simulink model "NewControlSim"  (R2024b)
settings: Solver=ode23s  StartTime=0.0  StopTime=173  RelTol=1e-3
values from neighbouring files (symbols this model uses):
  Af = 0.94    [new-sim-workspace.mat]    (also in workspace-var-complete-jan.mat; workspace_var_dec_2024.mat; workspace_var_jan_2024.mat)
  B = 10    [new-sim-workspace.mat]    (also in workspace-var-complete-jan.mat; workspace-vars.mat; workspace_var_dec_2024.mat; workspace_var_jan_2024.mat)
  C = 1.9    [new-sim-workspace.mat]    (also in workspace-var-complete-jan.mat; workspace-vars.mat; workspace_var_dec_2024.mat; workspace_var_jan_2024.mat)
  car_power_limit = 40    [new-sim-workspace.mat]    (also in workspace-var-complete-jan.mat)
  Cd = 0.94    [new-sim-workspace.mat]    (also in workspace-var-complete-jan.mat; workspace_var_dec_2024.mat; workspace_var_jan_2024.mat)
  cutoff_motor_temp = 90    [new-sim-workspace.mat]    (also in workspace-var-complete-jan.mat)
  D = 1    [new-sim-workspace.mat]    (also in workspace-var-complete-jan.mat; workspace-vars.mat; workspace_var_dec_2024.mat; workspace_var_jan_2024.mat)
  decrement_ratio_PL = 2.66666666667    [new-sim-workspace.mat]    (also in workspace-var-complete-jan.mat)
  g = 9.81    [new-sim-workspace.mat]    (also in workspace-var-complete-jan.mat; workspace-vars.mat; workspace_var_dec_2024.mat; workspace_var_jan_2024.mat)
  ideal_slip = 0.05    [new-sim-workspace.mat]    (also in workspace-var-complete-jan.mat)
  J_w = 0.5    [new-sim-workspace.mat]    (also in workspace-var-complete-jan.mat; workspace-vars.mat; workspace_var_dec_2024.mat; workspace_var_jan_2024.mat)
  M = 100    [new-sim-workspace.mat]    (also in workspace-var-complete-jan.mat; workspace-vars.mat; workspace_var_dec_2024.mat; workspace_var_jan_2024.mat)
  mass_den = 1.225    [new-sim-workspace.mat]    (also in workspace-var-complete-jan.mat; workspace_var_dec_2024.mat; workspace_var_jan_2024.mat)
  max_torque_req = 90    [new-sim-workspace.mat]    (also in workspace-var-complete-jan.mat)
  R = 0.5    [new-sim-workspace.mat]    (also in workspace-var-complete-jan.mat; workspace-vars.mat; workspace_var_dec_2024.mat; workspace_var_jan_2024.mat)
libraries: slpidlib x1
settings Model: Creator=shykizzy  LastModifiedBy=shykizzy

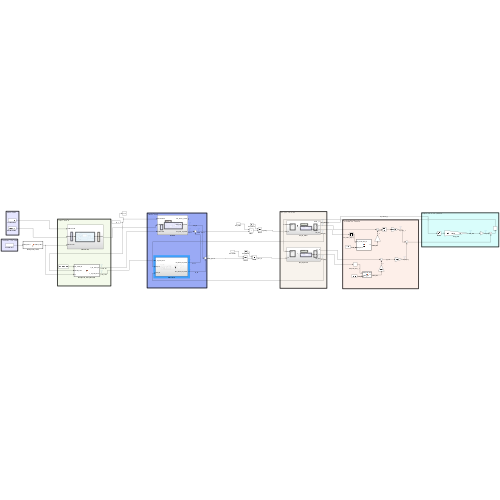
[thumbnail: Simulink's stored preview of the top-level diagram]
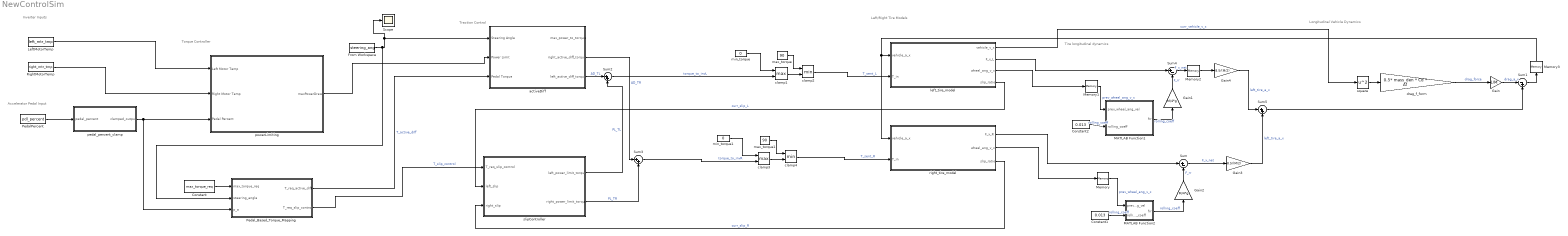
== system NewControlSim ==
  note: Longitudinal Vehicle Dynamics
  note: Traction Control
  note: Torque Controller
  note: Left/Right Tire Models
  note: Accelerator Pedal Input
  note: Inverter Inputs
  note: Tire longitudinal dynamics
  Constant : Constant  Value=max_torque_req
  Constant1 : Constant  Value=0.013
  Constant2 : Constant  Value=0.013
  From Workspace : FromWorkspace  VariableName=steering_ang
  Gain : Gain  Gain=1/M
  Gain1 : Gain  Gain=M/4*g
  Gain2 : Gain  Gain=M/4*g
  Gain3 : Gain  Gain=8.5/(M/2)
  Gain4 : Gain  Gain=8.5/(M/2)
  LeftMotorTemp : FromWorkspace  VariableName=left_mtr_tmp
  MATLAB Function1 : MATLAB Function  TreatAsAtomicUnit=on
  MATLAB Function2 : MATLAB Function  TreatAsAtomicUnit=on
  Memory{,1..3} (4 alike) : Memory
  PedalPercent : FromWorkspace  VariableName=pdl_percent
  Pedal_Based_Torque_Mapping : MATLAB Function  TreatAsAtomicUnit=on
  RightMotorTemp : FromWorkspace  VariableName=right_mtr_tmp
  Scope : Scope
  Sum : Sum  Inputs=|+-
  Sum1 : Sum  Inputs=|-+
  Sum2 : Sum  Inputs=|++
  Sum3 : Sum  Inputs=|++
  Sum4 : Sum  Inputs=|+-
  Sum5 : Sum  Inputs=|++
  activeDiff : Subsystem
  clamp1 : MinMax  Function=max  Inputs=2
  clamp2 : MinMax  Inputs=2
  clamp3 : MinMax  Function=max  Inputs=2
  clamp4 : MinMax  Inputs=2
  drag_f_form : Gain  Gain=0.5* mass_den * Cd * Af
  left_tire_model : Subsystem
  max_torque : Constant  Value=90
  max_torque1 : Constant  Value=90
  min_torque : Constant  Value=0
  min_torque1 : Constant  Value=0
  pedal_percent_clamp : MATLAB Function  TreatAsAtomicUnit=on
  powerLimiting : Subsystem
  right_tire_model : Subsystem
  slipController : Subsystem
  square : Math  Operator=square
  wires:
  Gain2/1 -> Sum/2  "F_rr"
  Constant1/1 -> MATLAB Function2/2(rolling_coeff)  "rolling_coeff"
  Sum/1 -> Gain3/1  "F_x_net"
  Memory/1 -> MATLAB Function2/1(prev_wheel_ang_vel)  "prev_wheel_ang_v_x"
  MATLAB Function2/1(frr) -> Gain2/1  "rolling_coeff"
  PedalPercent/1 -> pedal_percent_clamp/1(pedal_percent)
  pedal_percent_clamp/1(clamped_output) -> powerLimiting/3(Pedal Percent), Pedal_Based_Torque_Mapping/3(p_a)
  LeftMotorTemp/1 -> powerLimiting/1(Left Motor Temp)
  RightMotorTemp/1 -> powerLimiting/2(Right Motor Temp)
  From Workspace/1 -> activeDiff/1(Steering Angle), Scope/1, Pedal_Based_Torque_Mapping/2(steering_angle)
  slipController/1(left_power_limit_torque) -> Sum2/2  "PL_TL"
  activeDiff/3(left_active_diff_torque) -> Sum2/1  "AD_TL"
  activeDiff/2(right_active_diff_torque) -> Sum3/1  "AD_TR"
  slipController/2(right_power_limit_torque) -> Sum3/2  "PL_TR"
  Memory1/1 -> MATLAB Function1/1(prev_wheel_ang_vel)  "prev_wheel_ang_v_x"
  MATLAB Function1/1(frr) -> Gain1/1  "rolling_coeff"
  Sum4/1 -> Memory2/1  "F_x_net"
  Constant2/1 -> MATLAB Function1/2(rolling_coeff)  "rolling_coeff"
  Gain1/1 -> Sum4/2  "F_rr"
  left_tire_model/3(wheel_ang_v_x) -> Memory1/1
  right_tire_model/2(wheel_ang_v_x) -> Memory/1
  right_tire_model/1(F_x_R) -> Sum/1
  left_tire_model/2(F_x_L) -> Sum4/1
  Gain3/1 -> Sum5/2  "left_tire_a_x"
  Gain4/1 -> Sum5/1  "left_tire_a_x"
  Constant/1 -> Pedal_Based_Torque_Mapping/1(max_torque_req)
  Sum5/1 -> Sum1/2
  Sum1/1 -> Memory3/1
  left_tire_model/1(vehicle_v_x) -> square/1  "curr_vehicle_v_x"
  square/1 -> drag_f_form/1
  drag_f_form/1 -> Gain/1  "drag_force"
  Gain/1 -> Sum1/1  "drag_a_x"
  Memory2/1 -> Gain4/1
  Memory3/1 -> right_tire_model/1(vehicle_a_x), left_tire_model/1(vehicle_a_x)
  Pedal_Based_Torque_Mapping/1(T_req_active_diff) -> activeDiff/3(Pedal Torque)  "T_active_diff"
  Pedal_Based_Torque_Mapping/2(T_req_slip_control) -> slipController/1(T_req_slip_control)  "T_slip_control"
  powerLimiting/1(maxPowerDraw) -> activeDiff/2(Power Limit)
  min_torque/1 -> clamp1/1
  max_torque/1 -> clamp2/1
  clamp1/1 -> clamp2/2
  Sum2/1 -> clamp1/2  "torque_to_invL"
  clamp2/1 -> left_tire_model/2(T_in)  "T_sent_L"
  min_torque1/1 -> clamp3/1
  max_torque1/1 -> clamp4/1
  clamp3/1 -> clamp4/2
  Sum3/1 -> clamp3/2  "torque_to_invR"
  clamp4/1 -> right_tire_model/2(T_in)  "T_sent_R"
  left_tire_model/4(slip_ratio) -> slipController/2(left_slip)  "curr_slip_L"
  right_tire_model/3(slip_ratio) -> slipController/3(right_slip)  "curr_slip_R"

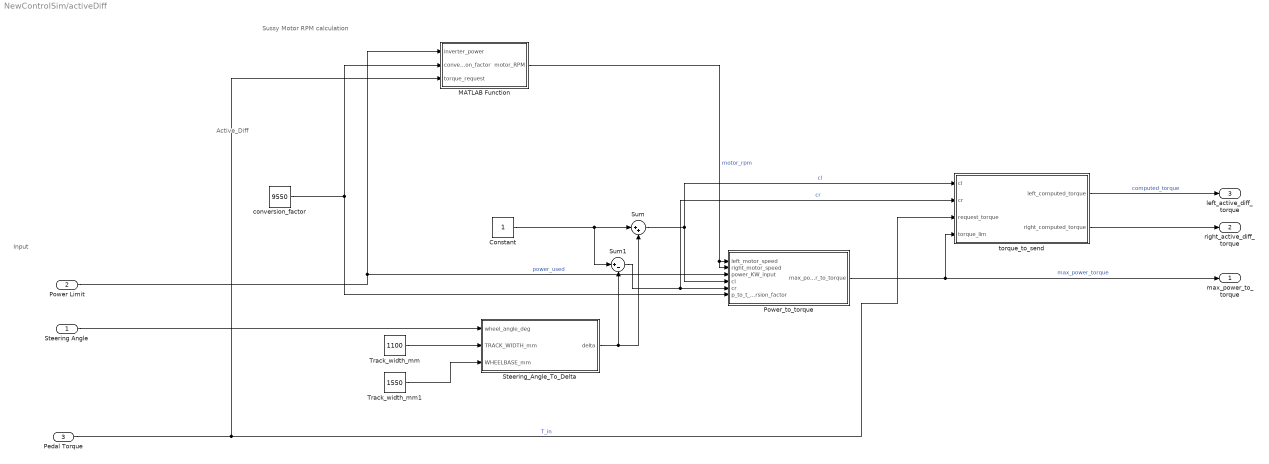
== system NewControlSim/activeDiff ==
  note: Input
  note: Active_Diff
  note: Sussy Motor RPM calculation
  Steering Angle : Inport
  Power Limit : Inport  Port=2
  Pedal Torque : Inport  Port=3
  Constant : Constant
  MATLAB Function : MATLAB Function  TreatAsAtomicUnit=on
  Power_to_torque : MATLAB Function  TreatAsAtomicUnit=on
  Steering_Angle_To_Delta : MATLAB Function  TreatAsAtomicUnit=on
  Sum : Sum  Inputs=|++
  Sum1 : Sum  Inputs=|+-
  Track_width_mm : Constant  Value=1100
  Track_width_mm1 : Constant  Value=1550
  conversion_factor : Constant  Value=9550
  torque_to_send : MATLAB Function  TreatAsAtomicUnit=on
  max_power_to_torque : Outport
  right_active_diff_torque : Outport  Port=2
  left_active_diff_torque : Outport  Port=3
  wires:
  Steering_Angle_To_Delta/1(delta) -> Sum1/2, Sum/2
  Pedal Torque/1 -> MATLAB Function/3(torque_request), torque_to_send/3(request_torque)  "T_in"
  Sum1/1 -> Power_to_torque/5(cr), torque_to_send/2(cr)  "cr"
  Constant/1 -> Sum1/1, Sum/1
  Steering Angle/1 -> Steering_Angle_To_Delta/1(wheel_angle_deg)
  Track_width_mm1/1 -> Steering_Angle_To_Delta/3(WHEELBASE_mm)
  Track_width_mm/1 -> Steering_Angle_To_Delta/2(TRACK_WIDTH_mm)
  MATLAB Function/1(motor_RPM) -> Power_to_torque/2(right_motor_speed), Power_to_torque/1(left_motor_speed)  "motor_rpm"
  conversion_factor/1 -> MATLAB Function/2(conversion_factor), Power_to_torque/6(p_to_t_conversion_factor)
  Sum/1 -> Power_to_torque/4(cl), torque_to_send/1(cl)  "cl"
  Power Limit/1 -> MATLAB Function/1(inverter_power), Power_to_torque/3(power_KW_input)  "power_used"
  Power_to_torque/1(max_power_to_torque) -> torque_to_send/4(torque_lim), max_power_to_torque/1  "max_power_torque"
  torque_to_send/1(left_computed_torque) -> left_active_diff_torque/1  "computed_torque"
  torque_to_send/2(right_computed_torque) -> right_active_diff_torque/1

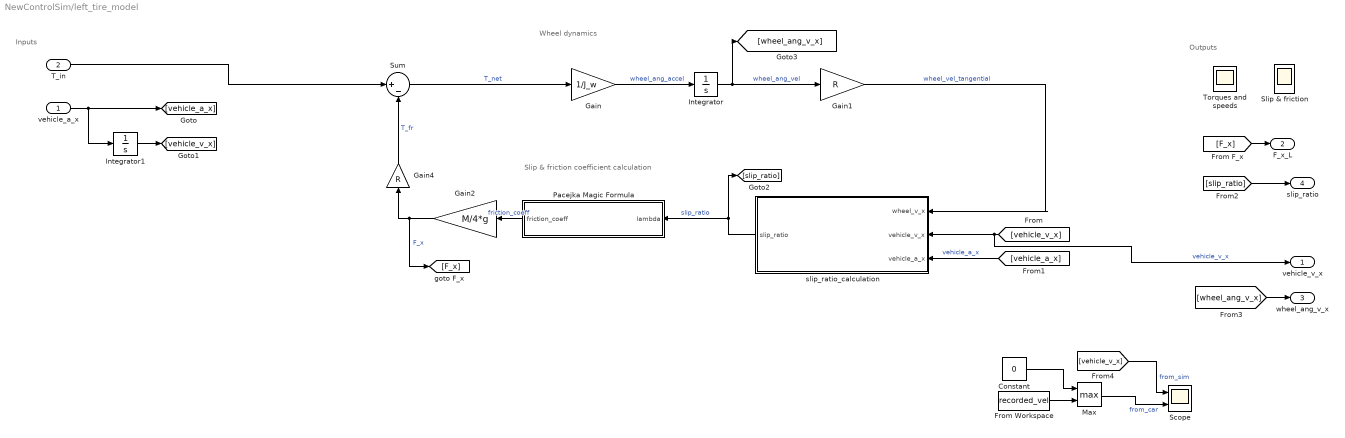
== system NewControlSim/left_tire_model ==
  note: Inputs
  note: Slip & friction coefficient calculation
  note: Wheel dynamics
  note: Outputs
  vehicle_a_x : Inport
  T_in : Inport  Port=2
  Constant : Constant  Value=0
  From Workspace : FromWorkspace  VariableName=recorded_vel  SampleTime=-1
  Gain : Gain  Gain=1/J_w
  Gain1 : Gain  Gain=R
  Gain2 : Gain  Gain=M/4*g
  Gain4 : Gain  Gain=R
  Integrator : Integrator
  Integrator1 : Integrator
  Max : MinMax  Function=max  Inputs=2
  Pacejka Magic Formula : MATLAB Function  TreatAsAtomicUnit=on
  Scope : Scope  NumInputPorts=2
  Slip & friction : Scope
      settings: Floating=on
  Sum : Sum  Inputs=|+-
  Torques and speeds : Scope
      settings: Floating=on
  slip_ratio_calculation : MATLAB Function  TreatAsAtomicUnit=on
  vehicle_v_x : Outport
  F_x_L : Outport  Port=2
  wheel_ang_v_x : Outport  Port=3
  slip_ratio : Outport  Port=4
  wires:
  Sum/1 -> Gain/1  "T_net"
  Gain1/1 -> slip_ratio_calculation/1(wheel_v_x)  "wheel_vel_tangential"
  Integrator/1 -> Gain1/1, [wheel_ang_v_x]  "wheel_ang_vel"
  Gain/1 -> Integrator/1  "wheel_ang_accel"
  slip_ratio_calculation/1(slip_ratio) -> Pacejka Magic Formula/1(lambda), [slip_ratio]  "slip_ratio"
  vehicle_a_x/1 -> Integrator1/1, [vehicle_a_x]
  Integrator1/1 -> [vehicle_v_x]
  [vehicle_v_x] -> slip_ratio_calculation/2(vehicle_v_x), vehicle_v_x/1  "vehicle_v_x"
  [vehicle_a_x] -> slip_ratio_calculation/3(vehicle_a_x)  "vehicle_a_x"
  [F_x] -> F_x_L/1
  [slip_ratio] -> slip_ratio/1
  Gain2/1 -> [F_x], Gain4/1  "F_x"
  Pacejka Magic Formula/1(friction_coeff) -> Gain2/1  "friction_coeff"
  Gain4/1 -> Sum/2  "T_fr"
  T_in/1 -> Sum/1
  [wheel_ang_v_x] -> wheel_ang_v_x/1
  From Workspace/1 -> Max/2
  Constant/1 -> Max/1
  Max/1 -> Scope/2  "from_car"
  [vehicle_v_x] -> Scope/1  "from_sim"

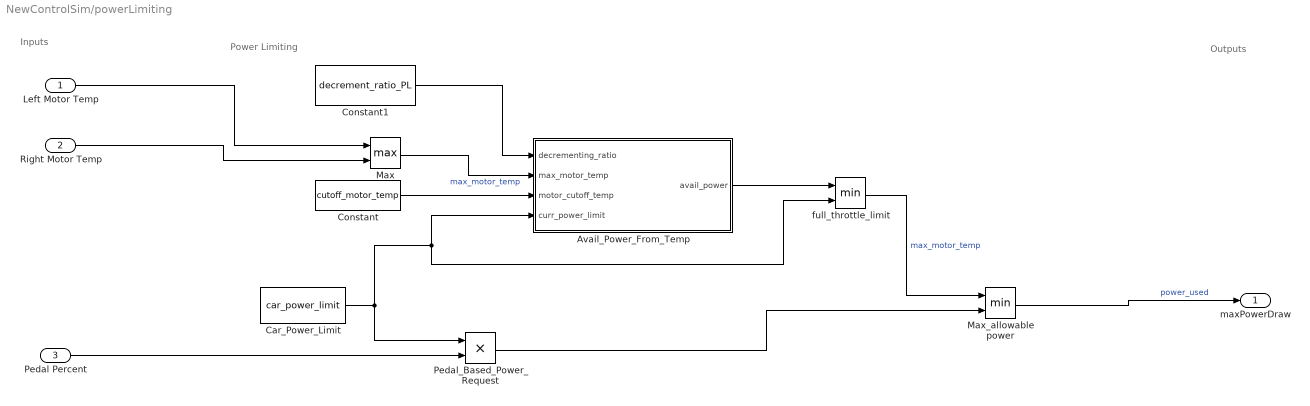
== system NewControlSim/powerLimiting ==
  note: Outputs
  note: Inputs
  note: Power Limiting
  Left Motor Temp : Inport
  Right Motor Temp : Inport  Port=2
  Pedal Percent : Inport  Port=3
  Avail_Power_From_Temp : MATLAB Function  TreatAsAtomicUnit=on
  Car_Power_Limit : Constant  Value=car_power_limit
  Constant : Constant  Value=cutoff_motor_temp
  Constant1 : Constant  Value=decrement_ratio_PL
  Max : MinMax  Function=max  Inputs=2
  Max_allowable power : MinMax  Inputs=2
  Pedal_Based_Power_Request : Product
  full_throttle_limit : MinMax  Inputs=2
  maxPowerDraw : Outport
  wires:
  Left Motor Temp/1 -> Max/1
  Car_Power_Limit/1 -> full_throttle_limit/2, Avail_Power_From_Temp/4(curr_power_limit), Pedal_Based_Power_Request/1
  Constant1/1 -> Avail_Power_From_Temp/1(decrementing_ratio)
  Pedal Percent/1 -> Pedal_Based_Power_Request/2
  Max/1 -> Avail_Power_From_Temp/2(max_motor_temp)  "max_motor_temp"
  Right Motor Temp/1 -> Max/2
  full_throttle_limit/1 -> Max_allowable power/1  "max_motor_temp"
  Avail_Power_From_Temp/1(avail_power) -> full_throttle_limit/1
  Pedal_Based_Power_Request/1 -> Max_allowable power/2
  Constant/1 -> Avail_Power_From_Temp/3(motor_cutoff_temp)
  Max_allowable power/1 -> maxPowerDraw/1  "power_used"

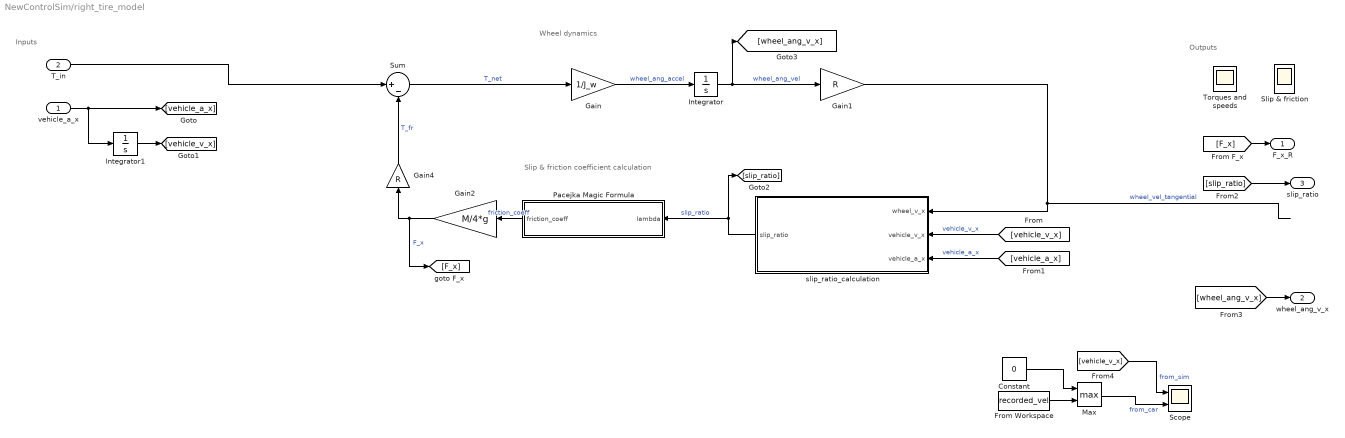
== system NewControlSim/right_tire_model ==
  note: Inputs
  note: Slip & friction coefficient calculation
  note: Wheel dynamics
  note: Outputs
  vehicle_a_x : Inport
  T_in : Inport  Port=2
  Constant : Constant  Value=0
  From Workspace : FromWorkspace  VariableName=recorded_vel  SampleTime=-1
  Gain : Gain  Gain=1/J_w
  Gain1 : Gain  Gain=R
  Gain2 : Gain  Gain=M/4*g
  Gain4 : Gain  Gain=R
  Integrator : Integrator
  Integrator1 : Integrator
  Max : MinMax  Function=max  Inputs=2
  Pacejka Magic Formula : MATLAB Function  TreatAsAtomicUnit=on
  Scope : Scope  NumInputPorts=2
  Slip & friction : Scope
      settings: Floating=on
  Sum : Sum  Inputs=|+-
  Torques and speeds : Scope
      settings: Floating=on
  slip_ratio_calculation : MATLAB Function  TreatAsAtomicUnit=on
  F_x_R : Outport
  wheel_ang_v_x : Outport  Port=2
  slip_ratio : Outport  Port=3
  wires:
  Sum/1 -> Gain/1  "T_net"
  Gain1/1 -> slip_ratio_calculation/1(wheel_v_x)  "wheel_vel_tangential"
  Integrator/1 -> Gain1/1, [wheel_ang_v_x]  "wheel_ang_vel"
  Gain/1 -> Integrator/1  "wheel_ang_accel"
  slip_ratio_calculation/1(slip_ratio) -> Pacejka Magic Formula/1(lambda), [slip_ratio]  "slip_ratio"
  vehicle_a_x/1 -> Integrator1/1, [vehicle_a_x]
  Integrator1/1 -> [vehicle_v_x]
  [vehicle_v_x] -> slip_ratio_calculation/2(vehicle_v_x)  "vehicle_v_x"
  [vehicle_a_x] -> slip_ratio_calculation/3(vehicle_a_x)  "vehicle_a_x"
  [F_x] -> F_x_R/1
  [slip_ratio] -> slip_ratio/1
  Gain2/1 -> [F_x], Gain4/1  "F_x"
  Pacejka Magic Formula/1(friction_coeff) -> Gain2/1  "friction_coeff"
  Gain4/1 -> Sum/2  "T_fr"
  T_in/1 -> Sum/1
  [wheel_ang_v_x] -> wheel_ang_v_x/1
  From Workspace/1 -> Max/2
  Constant/1 -> Max/1
  Max/1 -> Scope/2  "from_car"
  [vehicle_v_x] -> Scope/1  "from_sim"

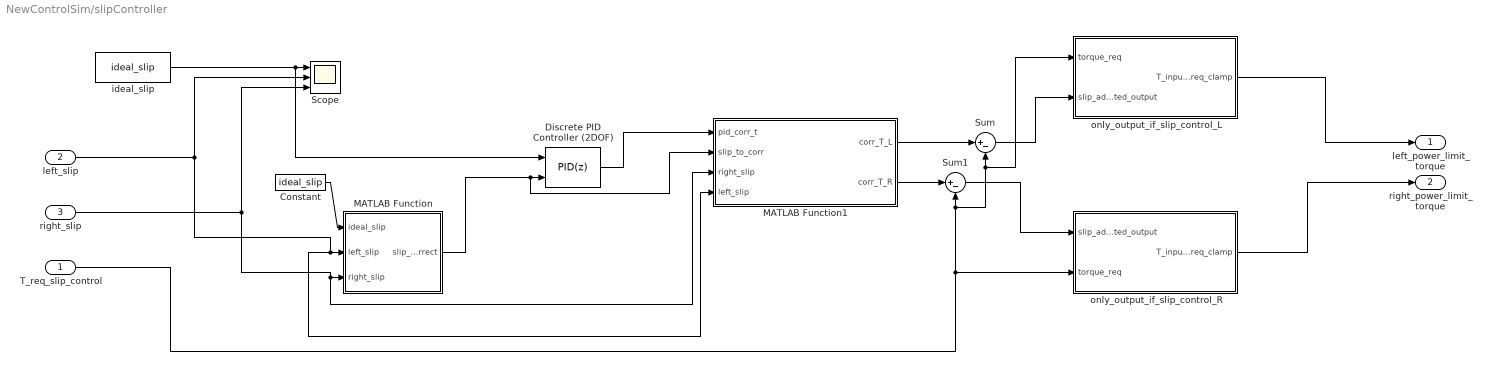
== system NewControlSim/slipController ==
  T_req_slip_control : Inport
  left_slip : Inport  Port=2
  right_slip : Inport  Port=3
  Constant : Constant  Value=ideal_slip
  Discrete PID Controller (2DOF) : slpidlib/PID Controller (2DOF)  Controller=PID  Form=Parallel  TimeDomain=Discrete-time  UseExternalTs=off  SampleTime=-1  IntegratorMethod=Forward Euler  FilterMethod=Forward Euler  ControllerParametersSource=internal  P=1  I=0  UseKiTs=off  D=0  UseExternalDerivativeSource=off  N=100  UseFilter=on  b=1  c=1  TunerSelectOption=Transfer Function Based (PID Tuner App)  InitialConditionSource=internal  InitialConditionForIntegrator=0  InitialConditionForFilter=0  DifferentiatorICPrevScaledInput=0  ExternalReset=none  TrackingMode=off  Kt=1  LimitOutput=off  SatLimitsSource=internal  UpperSaturationLimit=inf  LowerSaturationLimit=-inf  LinearizeAsGain=off  AntiWindupMode=none  Kb=1  LimitIntegrator=off  UpperIntegratorSaturationLimit=inf  LowerIntegratorSaturationLimit=-inf  POutMin=[]  POutMax=[]  IOutMin=[]  IOutMax=[]  DOutMin=[]  DOutMax=[]  NOutMin=[]  NOutMax=[]  bOutMin=[]  bOutMax=[]  cOutMin=[]  cOutMax=[]  SumOutMin=[]  SumOutMax=[]  SaturationOutMin=[]  SaturationOutMax=[]  PParamMin=[]  PParamMax=[]  IParamMin=[]  IParamMax=[]  DParamMin=[]  DParamMax=[]  NParamMin=[]  NParamMax=[]  bParamMin=[]  bParamMax=[]  cParamMin=[]  cParamMax=[]  KbParamMin=[]  KbParamMax=[]  KtParamMin=[]  KtParamMax=[]  KbOutMin=[]  KbOutMax=[]  KtOutMin=[]  KtOutMax=[]  IntegratorOutMin=[]  IntegratorOutMax=[]  FilterOutMin=[]  FilterOutMax=[]  SumI1OutMin=[]  SumI1OutMax=[]  SumI2OutMin=[]  SumI2OutMax=[]  SumI3OutMin=[]  SumI3OutMax=[]  SumI4OutMin=[]  SumI4OutMax=[]  SumDOutMin=[]  SumDOutMax=[]  Sum1OutMin=[]  Sum1OutMax=[]  Sum2OutMin=[]  Sum2OutMax=[]  Sum3OutMin=[]  Sum3OutMax=[]  DifferentiatorOutMin=[]  DifferentiatorOutMax=[]  FilterDiffOutCoefMin=[]  FilterDiffOutCoefMax=[]  ReciprocalOutMin=[]  ReciprocalOutMax=[]  SumDenOutMin=[]  SumDenOutMax=[]  SumNumOutMin=[]  SumNumOutMax=[]  DivideOutMin=[]  DivideOutMax=[]  UdiffTsProdOutMin=[]  UdiffTsProdOutMax=[]  NTsProdOutMin=[]  NTsProdOutMax=[]  UintegralTsProdOutMin=[]  UintegralTsProdOutMax=[]  UngainTsProdOutMin=[]  UngainTsProdOutMax=[]  ClampingZeroOutDataTypeStr=Inherit: Inherit via back propagation  ClampingZeroOutMin=[]  ClampingZeroOutMax=[]  FilterDenConstantOutDataTypeStr=Inherit: Inherit via back propagation  FilterDenConstantOutMin=[]  FilterDenConstantOutMax=[]  PCopyOutDataTypeStr=Inherit: Inherit via back propagation  PCopyOutMin=[]  PCopyOutMax=[]  NCopyOutDataTypeStr=Inherit: Inherit via back propagation  NCopyOutMin=[]  NCopyOutMax=[]  IntegratorContinuousStateAttributes=''  IntegratorStateMustResolveToSignalObject=off  IntegratorRTWStateStorageClass=Auto  FilterContinuousStateAttributes=''  FilterStateMustResolveToSignalObject=off  FilterRTWStateStorageClass=Auto  ParallelPVariant=InternalParameters  IdealPVariant=Disabled  IVariant=InternalParameters  DVariant=InternalParameters  bVariant=InternalParameters  cVariant=InternalParameters  IntegratorVariant=Discrete  SatVariant=Disabled  AWVariant=Passthrough  PCopyVariant=Disabled  TRVariant=Disabled  FdbkBlocksVariant=Forward  IdealPFdbkVariant=Disabled  SatFdbkVariant=Disabled  DerivativeFilterVariant=ForwardEulerFilter  NVariant=InternalParameters  NCopyVariant=Disabled  FilterICVariant=InternalICsFilter  IntegratorICVariant=InternalICs  ExternalResetVariant=Disabled  TRSumVariant=Passthrough  SumFdbkVariant=Disabled  SumVariant=Sum_PID  TsampFilterVariant=InternalTs  TsampNgainVariant=Passthrough  TsampIntegralVariant=Disabled_SignalSpec  ExternalSaturationOutDataTypeStr=Inherit: Same as second input  DerivativeSourceVariant=ErrorSignal  PreIntVariant=InternalPreInt
      settings: LibrarySourceBlock=simulink/Discrete/Discrete PID Controller (2DOF)
  MATLAB Function : MATLAB Function  TreatAsAtomicUnit=on
  MATLAB Function1 : MATLAB Function  TreatAsAtomicUnit=on
  Scope : Scope  NumInputPorts=3
  Sum : Sum  Inputs=|+-
  Sum1 : Sum  Inputs=|+-
  ideal_slip : Constant  Value=ideal_slip
  only_output_if_slip_control_L : MATLAB Function  TreatAsAtomicUnit=on
  only_output_if_slip_control_R : MATLAB Function  TreatAsAtomicUnit=on
  left_power_limit_torque : Outport
  right_power_limit_torque : Outport  Port=2
  wires:
  ideal_slip/1 -> Scope/1, Discrete PID Controller (2DOF)/1
  left_slip/1 -> MATLAB Function1/4(left_slip), MATLAB Function/2(left_slip), Scope/2
  right_slip/1 -> MATLAB Function1/3(right_slip), MATLAB Function/3(right_slip), Scope/3
  MATLAB Function/1(slip_to_correct) -> MATLAB Function1/2(slip_to_corr), Discrete PID Controller (2DOF)/2
  Discrete PID Controller (2DOF)/1 -> MATLAB Function1/1(pid_corr_t)
  MATLAB Function1/1(corr_T_L) -> Sum/1
  MATLAB Function1/2(corr_T_R) -> Sum1/1
  Constant/1 -> MATLAB Function/1(ideal_slip)
  Sum/1 -> only_output_if_slip_control_L/2(slip_adjusted_output)
  Sum1/1 -> only_output_if_slip_control_R/1(slip_adjusted_output)
  T_req_slip_control/1 -> only_output_if_slip_control_R/2(torque_req), only_output_if_slip_control_L/1(torque_req), Sum/2, Sum1/2
  only_output_if_slip_control_R/1(T_input_req_clamp) -> right_power_limit_torque/1
  only_output_if_slip_control_L/1(T_input_req_clamp) -> left_power_limit_torque/1

== matlab function NewControlSim/pedal_percent_clamp ==
  data: pedal_percent input; clamped_output output
function clamped_output = fcn(pedal_percent)

if pedal_percent < 0
    clamped_output = 0;

elseif pedal_percent > 1
    clamped_output = 1;

else
    clamped_output = pedal_percent;
    
end

== matlab function NewControlSim/right_tire_model/slip_ratio_calculation ==
  data: wheel_v_x input; slip_ratio output; vehicle_v_x input; TOL parameter; vehicle_a_x input
function slip_ratio = fcn(wheel_v_x, vehicle_v_x, TOL, vehicle_a_x)
% This is derived from pg. 100 of Rajamani - Vehicle Dynamics and Control
% (2006)

if vehicle_a_x >= 0
    slip_ratio = (wheel_v_x- vehicle_v_x)/(wheel_v_x + TOL);
else
    slip_ratio = (wheel_v_x - vehicle_v_x)/(vehicle_v_x + TOL);
end

== matlab function NewControlSim/MATLAB Function1 ==
  data: prev_wheel_ang_vel input; frr output; rolling_coeff input
function frr = fcn(prev_wheel_ang_vel, rolling_coeff)

% no physics formula to refer for this however I did this based on
% intuition... essentially I don't believe rolling resistance should be
% effecting the friction force on the car if the wheels are not moving

if(prev_wheel_ang_vel <= 0)
    frr = 0;
else
    frr = rolling_coeff; 
end

== matlab function NewControlSim/MATLAB Function2 ==
  data: prev_wheel_ang_vel input; frr output; rolling_coeff input
function frr = fcn(prev_wheel_ang_vel, rolling_coeff)

% no physics formula to refer for this however I did this based on
% intuition... essentially I don't believe rolling resistance should be
% effecting the friction force on the car if the wheels are not moving

if(prev_wheel_ang_vel <= 0)
    frr = 0;
else
    frr = rolling_coeff; 
end

== matlab function NewControlSim/slipController/MATLAB Function ==
  data: ideal_slip input; left_slip input; slip_to_correct output; right_slip input
function slip_to_correct = fcn(ideal_slip, left_slip, right_slip)

error_left = abs(left_slip - ideal_slip)
error_right = abs(right_slip - ideal_slip)

if error_left <= error_right
    slip_to_correct = left_slip
else
    slip_to_correct = right_slip
end

== matlab function NewControlSim/left_tire_model/Pacejka Magic Formula ==
  data: lambda input double size=1; friction_coeff output double size=1; B parameter double size=1; C parameter double size=1; D parameter double size=1; E parameter double size=1
function friction_coeff = fcn(lambda, B, C, D, E)

friction_coeff = D*sin(C*atan(B*lambda -  E*(B*lambda - atan(B*lambda))));

== matlab function NewControlSim/slipController/MATLAB Function1 ==
  data: pid_corr_t input; corr_T_L output; slip_to_corr input; right_slip input; left_slip input; corr_T_R output
function [corr_T_L, corr_T_R] = fcn(pid_corr_t, ...
    slip_to_corr, right_slip,left_slip)

% This function is there to route the PID correction based on which motor
% ie. wheel the correction is for. The other wheel should recieve a 0
% correction

corr_T_L = 0;
corr_T_R = 0; 

if(slip_to_corr == left_slip)
    corr_T_L = pid_corr_t
elseif (slip_to_corr == right_slip)
    corr_T_R = pid_corr_t
end

== matlab function NewControlSim/slipController/only_output_if_slip_control_L ==
  data: torque_req input; T_input_req_clamp output; slip_adjusted_output input
function T_input_req_clamp = fcn(torque_req, slip_adjusted_output)

if torque_req == 0
    T_input_req_clamp = slip_adjusted_output;
else
    T_input_req_clamp = 0;
end

== matlab function NewControlSim/slipController/only_output_if_slip_control_R ==
  data: slip_adjusted_output input; torque_req input; T_input_req_clamp output
function T_input_req_clamp = fcn(slip_adjusted_output, torque_req)

if torque_req == 0
    T_input_req_clamp = slip_adjusted_output;
else
    T_input_req_clamp = 0;
end

== matlab function NewControlSim/left_tire_model/slip_ratio_calculation ==
  data: wheel_v_x input; slip_ratio output; vehicle_v_x input; TOL parameter; vehicle_a_x input
function slip_ratio = fcn(wheel_v_x, vehicle_v_x, TOL, vehicle_a_x)
% This is derived from pg. 100 of Rajamani - Vehicle Dynamics and Control
% (2006)

if vehicle_a_x >= 0
    slip_ratio = (wheel_v_x- vehicle_v_x)/(wheel_v_x + TOL);
else
    slip_ratio = (wheel_v_x - vehicle_v_x)/(vehicle_v_x + TOL);
end

== matlab function NewControlSim/powerLimiting/Avail_Power_From_Temp ==
  data: decrementing_ratio input; max_motor_temp input; avail_power output; motor_cutoff_temp input; curr_power_limit input
function avail_power = fcn( decrementing_ratio,max_motor_temp, ...
    motor_cutoff_temp, curr_power_limit)

avail_power = curr_power_limit;

if (max_motor_temp - motor_cutoff_temp) >= 30.0
    avail_power = 0.0;
elseif max_motor_temp > motor_cutoff_temp
    avail_power = curr_power_limit - ...
    (max_motor_temp - motor_cutoff_temp) * ...
    decrementing_ratio;
end

== matlab function NewControlSim/right_tire_model/Pacejka Magic Formula ==
  data: lambda input double size=1; friction_coeff output double size=1; B parameter double size=1; C parameter double size=1; D parameter double size=1; E parameter double size=1
function friction_coeff = fcn(lambda, B, C, D, E)

friction_coeff = D*sin(C*atan(B*lambda -  E*(B*lambda - atan(B*lambda))));

== matlab function NewControlSim/activeDiff/torque_to_send ==
  data: left_computed_torque output; cl input; cr input; request_torque input; torque_lim input; right_computed_torque output
% this block should theoritically not do anything as of now because of the
% way motor speed was calculate (the output of maxPower_to_Torque is going
% to be requested torque as of now)

function [left_computed_torque, right_computed_torque]...
= fcn(cl, cr, request_torque, torque_lim)

% will be the same for now 
torque_left_nm = request_torque * cl; 
torque_right_nm = request_torque * cr; 

scale = 1.0; 
torque_req_max = max([torque_left_nm, torque_right_nm]);

if torque_req_max > torque_lim 
    scale = torque_lim / torque_req_max;
end 
% same implementation as code, essentially the idea is that if we scale
% does the larger torque to torque_lim in the case of torque_req_max > than
% torque_lim then applying the same scale to the other wheel's torque will
% preserve the ratio that was previously set by CL and CR 
left_computed_torque = torque_left_nm * scale;
right_computed_torque = torque_right_nm * scale;

== matlab function NewControlSim/activeDiff/Steering_Angle_To_Delta ==
  data: wheel_angle_deg input; TRACK_WIDTH_mm input; WHEELBASE_mm input; delta output
function delta = fcn(wheel_angle_deg, TRACK_WIDTH_mm, WHEELBASE_mm)

delta = TRACK_WIDTH_mm * tan(deg2rad(wheel_angle_deg)) / (2 * WHEELBASE_mm);

== matlab function NewControlSim/activeDiff/Power_to_torque ==
  data: left_motor_speed input; right_motor_speed input; power_KW_input input; cl input; max_power_to_torque output; cr input; p_to_t_conversion_factor input
function max_power_to_torque = fcn(left_motor_speed, right_motor_speed,power_KW_input, ...
    cl,cr, p_to_t_conversion_factor)

% taken directly from code .. standard motor torque charac eqn assumes
% torque is equally distributed between left and right wheel

% since our power limit torque is calcuated using requested torque if we
% use the main power to torque formula that we use in code we will always
% get half of the requested torque as the limit and there fore the output
% torque will be defaulted to the power limit... good thing is that this
% shows that the defaulting if power limit torque exceeded works bad thing
% is that we are straying away from our actual mathematical model...
% tentatively I have changed the calculation for power to torque from power
% limit to only account for 1 wheel as this is a one wheel model

max_power_to_torque = (p_to_t_conversion_factor * power_KW_input)/ ...
(left_motor_speed + 0.00001);

== matlab function NewControlSim/Pedal_Based_Torque_Mapping ==
  data: max_torque_req input; steering_angle input; p_a input; T_req_active_diff output; T_req_slip_control output
function [T_req_active_diff, T_req_slip_control]= ...
fcn(max_torque_req,steering_angle, p_a)



if (-10.0 <= steering_angle && steering_angle <= 10.0)
    T_req_active_diff = 0;
    T_req_slip_control = max_torque_req* p_a;
else 
    T_req_active_diff = max_torque_req * p_a;
    T_req_slip_control = 0;
end

== matlab function NewControlSim/activeDiff/MATLAB Function ==
  data: inverter_power input; conversion_factor input; torque_request input; motor_RPM output
function motor_RPM = fcn(inverter_power, conversion_factor, torque_request)

% kinda sus calculation but we need a way to calculate motor speed from
% torque... decided to use W = 9550 * P in KW /T N in rpm 
% problem is the power_to_torque function just calculates using the same
% formula so essentially it will go back to the torque request 

motor_RPM = (inverter_power * conversion_factor) / (torque_request + 0.00001);
